simulink library "NeuroModelerLibrary"  (Simulink 10.2)
settings: Solver=ode45  StartTime=0.0  StopTime=10.0  RelTol=1e-3
libraries: $bdroot x672, simulink x5, neural x2
(part 4 of 5)

== system NeuroModelerLibrary/Sized Cells/CSNM4x3 ==
  Stimulate1 : Inport
  Stimulate2 : Inport  Port=2
  Stimulate3 : Inport  Port=3
  Stimulate4 : Inport  Port=4
  Arresting1 : Inport  Port=5
  Arresting2 : Inport  Port=6
  Arresting3 : Inport  Port=7
  Arresting4 : Inport  Port=8
  C1 : Constant
  C2 : Constant  Value=0.93
  C3 : Constant  Value=-1
  CSNM Compartment{,1..6} (7 alike) : $bdroot/Neuron Elements/CSNM Compartment  ACm=1e-9  ARm=1e7  ECm=1e-9  ERm=1e7  ARFm=1e7  ERFm=1e7  U0=-0.070  sign=-1
  CSNM LTZone : $bdroot/Neuron Elements/CSNM LTZone  NM=1  FB=2  T=-0.055  switchOff=-0.1
  CSNM Synapse{,1..7} (8 alike) : $bdroot/Neuron Elements/CSNM Synapse  SecretionTC=0.001  DecompositionTC=0.005  UseKsi=off  Rs=2e7  ksi=1  U0=-0.070  Weight=1  sign=off
  Sum7 : Sum  Inputs=++++++++  InputSameDT=on  SaturateOnIntegerOverflow=on  OutDataTypeStr=Inherit: Same as first input
  Out : Outport  VectorParamsAs1DForOutWhenUnconnected=off
  Visual : Outport  Port=2  VectorParamsAs1DForOutWhenUnconnected=off
  Potential : Outport  Port=3  VectorParamsAs1DForOutWhenUnconnected=off
  wires:
  CSNM Synapse7/1 -> CSNM Compartment/5
  Arresting4/1 -> CSNM Synapse7/1
  CSNM Synapse6/1 -> CSNM Compartment4/5
  Arresting3/1 -> CSNM Synapse6/1
  CSNM Synapse5/1 -> CSNM Compartment5/5
  Arresting2/1 -> CSNM Synapse5/1
  Stimulate4/1 -> CSNM Synapse/1
  CSNM Synapse/1 -> CSNM Compartment/1
  Stimulate3/1 -> CSNM Synapse1/1
  CSNM Synapse1/1 -> CSNM Compartment4/1
  Stimulate2/1 -> CSNM Synapse2/1
  CSNM Synapse2/1 -> CSNM Compartment5/1
  CSNM Synapse3/1 -> CSNM Compartment6/1
  CSNM Synapse4/1 -> CSNM Compartment6/5
  CSNM Compartment6/2 -> CSNM Compartment5/4
  CSNM Compartment6/1 -> CSNM Compartment5/2
  CSNM Compartment5/2 -> CSNM Compartment4/4
  CSNM Compartment5/1 -> CSNM Compartment4/2
  CSNM LTZone/4 -> Visual/1
  CSNM LTZone/1 -> Out/1
  C1/1 -> CSNM LTZone/2
  Stimulate1/1 -> CSNM Synapse3/1
  Arresting1/1 -> CSNM Synapse4/1
  C2/1 -> CSNM Compartment1/2, CSNM Compartment3/2, CSNM Compartment2/2, CSNM Compartment6/2
  C3/1 -> CSNM Compartment6/4, CSNM Compartment1/4, CSNM Compartment3/4, CSNM Compartment2/4
  Sum7/1 -> CSNM LTZone/1
  CSNM LTZone/3 -> CSNM Compartment/3, CSNM Compartment1/3, CSNM Compartment3/3, CSNM Compartment2/3
  CSNM Compartment/1 -> Sum7/1
  CSNM Compartment/2 -> Sum7/2
  CSNM LTZone/2 -> Potential/1
  CSNM Compartment1/1 -> Sum7/3
  CSNM Compartment1/2 -> Sum7/4
  CSNM Compartment2/1 -> Sum7/5
  CSNM Compartment2/2 -> Sum7/6
  CSNM Compartment3/1 -> Sum7/7
  CSNM Compartment3/2 -> Sum7/8
  CSNM Compartment4/2 -> CSNM Compartment/4
  CSNM Compartment4/1 -> CSNM Compartment/2

== system NeuroModelerLibrary/Sized Cells/Cell IaF 1x4 ==
  Stimulate1 : Inport
  Stimulate2 : Inport  Port=2
  Stimulate3 : Inport  Port=3
  Stimulate4 : Inport  Port=4
  CSNM Synapse{40..43} (4 alike) : $bdroot/Neuron Elements/CSNM Synapse  SecretionTC=0.001  DecompositionTC=0.005  UseKsi=off  Rs=2e7  ksi=1  U0=-0.070  Weight=1  sign=off
  Constant6 : Constant  Value=-0.070
  IaF LTZone6 : Subsystem  mask{tau_m=0.01, Cm=250e-12, I_const=0, E_L=-0.070, V_reset=-0.10, V_th=-0.055}
      mask prompts: tau_m "Membrane time constatnt"; Cm "Membrane capacity"; I_const "Constant input current"; E_L "Resting membrane potential"; V_reset "Reset membrane potential"; V_th "Threshold potential"
  IaF Membrane Segment18 : Subsystem  mask{tau_m=0.01, Cm=250e-12, I_const=0, E_L=-0.070, V_reset=-0.10, V_th=-0.055}
      mask prompts: tau_m "Membrane time constatnt"; Cm "Membrane capacity"; I_const "Constant input current"; E_L "Resting membrane potential"; V_reset "Reset membrane potential"; V_th "Threshold potential"
  IaF Membrane Segment19 : Subsystem  mask{tau_m=0.01, Cm=250e-12, I_const=0, E_L=-0.070, V_reset=-0.10, V_th=-0.055}
      mask prompts: tau_m "Membrane time constatnt"; Cm "Membrane capacity"; I_const "Constant input current"; E_L "Resting membrane potential"; V_reset "Reset membrane potential"; V_th "Threshold potential"
  IaF Membrane Segment20 : Subsystem  mask{tau_m=0.01, Cm=250e-12, I_const=0, E_L=-0.070, V_reset=-0.10, V_th=-0.055}
      mask prompts: tau_m "Membrane time constatnt"; Cm "Membrane capacity"; I_const "Constant input current"; E_L "Resting membrane potential"; V_reset "Reset membrane potential"; V_th "Threshold potential"
  IaF Membrane Segment21 : Subsystem  mask{tau_m=0.01, Cm=250e-12, I_const=0, E_L=-0.070, V_reset=-0.10, V_th=-0.055}
      mask prompts: tau_m "Membrane time constatnt"; Cm "Membrane capacity"; I_const "Constant input current"; E_L "Resting membrane potential"; V_reset "Reset membrane potential"; V_th "Threshold potential"
  Potential : Outport
  wires:
  IaF Membrane Segment21/1(Out1) -> IaF Membrane Segment20/2(Resting Potential)
  IaF Membrane Segment20/1(Out1) -> IaF Membrane Segment19/2(Resting Potential)
  IaF Membrane Segment19/1(Out1) -> IaF Membrane Segment18/2(Resting Potential)
  CSNM Synapse41/1 -> IaF Membrane Segment20/1(Synapses)
  IaF LTZone6/1(Out) -> IaF Membrane Segment18/3(Reset Signal)  "Out"
  IaF Membrane Segment18/1(Out1) -> IaF LTZone6/1(Potential)  "IaF синапс + IaF нейрон"
  Constant6/1 -> IaF Membrane Segment21/2(Resting Potential)
  CSNM Synapse40/1 -> IaF Membrane Segment21/1(Synapses)
  Stimulate4/1 -> CSNM Synapse40/1
  CSNM Synapse43/1 -> IaF Membrane Segment18/1(Synapses)
  CSNM Synapse42/1 -> IaF Membrane Segment19/1(Synapses)
  Stimulate3/1 -> CSNM Synapse41/1
  IaF LTZone6/2(Out Potential) -> Potential/1
  Stimulate1/1 -> CSNM Synapse43/1
  Stimulate2/1 -> CSNM Synapse42/1

== system NeuroModelerLibrary/Sized Cells/Cell IaF 1x4-Syn4 ==
  Stimulate1 : Inport
  Stimulate2 : Inport  Port=2
  Stimulate3 : Inport  Port=3
  Stimulate4 : Inport  Port=4
  CSNM Synapse{8..11} (4 alike) : $bdroot/Neuron Elements/CSNM Synapse  SecretionTC=0.001  DecompositionTC=0.005  UseKsi=off  Rs=2e7  ksi=1  U0=-0.070  Weight=1  sign=off
  Constant4 : Constant  Value=-0.070
  IaF LTZone1 : Subsystem  mask{tau_m=0.01, Cm=250e-12, I_const=0, E_L=-0.070, V_reset=-0.10, V_th=-0.055}
      mask prompts: tau_m "Membrane time constatnt"; Cm "Membrane capacity"; I_const "Constant input current"; E_L "Resting membrane potential"; V_reset "Reset membrane potential"; V_th "Threshold potential"
  IaF Membrane Segment1 : Subsystem  mask{tau_m=0.01, Cm=250e-12, I_const=0, E_L=-0.070, V_reset=-0.10, V_th=-0.055}
      mask prompts: tau_m "Membrane time constatnt"; Cm "Membrane capacity"; I_const "Constant input current"; E_L "Resting membrane potential"; V_reset "Reset membrane potential"; V_th "Threshold potential"
  IaF Membrane Segment2 : Subsystem  mask{tau_m=0.01, Cm=250e-12, I_const=0, E_L=-0.070, V_reset=-0.10, V_th=-0.055}
      mask prompts: tau_m "Membrane time constatnt"; Cm "Membrane capacity"; I_const "Constant input current"; E_L "Resting membrane potential"; V_reset "Reset membrane potential"; V_th "Threshold potential"
  IaF Membrane Segment3 : Subsystem  mask{tau_m=0.01, Cm=250e-12, I_const=0, E_L=-0.070, V_reset=-0.10, V_th=-0.055}
      mask prompts: tau_m "Membrane time constatnt"; Cm "Membrane capacity"; I_const "Constant input current"; E_L "Resting membrane potential"; V_reset "Reset membrane potential"; V_th "Threshold potential"
  IaF Membrane Segment4 : Subsystem  mask{tau_m=0.01, Cm=250e-12, I_const=0, E_L=-0.070, V_reset=-0.10, V_th=-0.055}
      mask prompts: tau_m "Membrane time constatnt"; Cm "Membrane capacity"; I_const "Constant input current"; E_L "Resting membrane potential"; V_reset "Reset membrane potential"; V_th "Threshold potential"
  Sum2 : Sum  Inputs=++++  InputSameDT=on  SaturateOnIntegerOverflow=on  OutDataTypeStr=Inherit: Same as first input
  Potential : Outport
  wires:
  Sum2/1 -> IaF Membrane Segment4/1(Synapses)
  CSNM Synapse8/1 -> Sum2/1
  CSNM Synapse9/1 -> Sum2/2
  IaF Membrane Segment4/1(Out1) -> IaF Membrane Segment3/2(Resting Potential)
  Stimulate1/1 -> CSNM Synapse8/1
  Constant4/1 -> IaF Membrane Segment4/2(Resting Potential)
  IaF Membrane Segment2/1(Out1) -> IaF Membrane Segment1/2(Resting Potential)
  CSNM Synapse10/1 -> Sum2/3
  IaF Membrane Segment1/1(Out1) -> IaF LTZone1/1(Potential)  "IaF синапс + IaF нейрон"
  CSNM Synapse11/1 -> Sum2/4
  IaF LTZone1/2(Out Potential) -> Potential/1  "1 syn"
  IaF Membrane Segment3/1(Out1) -> IaF Membrane Segment2/2(Resting Potential)
  IaF LTZone1/1(Out) -> IaF Membrane Segment1/3(Reset Signal)  "Out"
  Stimulate2/1 -> CSNM Synapse9/1
  Stimulate3/1 -> CSNM Synapse10/1
  Stimulate4/1 -> CSNM Synapse11/1

== system NeuroModelerLibrary/Sized Cells/Cell IaF 2x4 ==
  Stimulate1 : Inport
  Stimulate2 : Inport  Port=2
  Stimulate3 : Inport  Port=3
  Stimulate4 : Inport  Port=4
  CSNM Synapse{40..43} (4 alike) : $bdroot/Neuron Elements/CSNM Synapse  SecretionTC=0.001  DecompositionTC=0.005  UseKsi=off  Rs=2e7  ksi=1  U0=-0.070  Weight=1  sign=off
  Constant7 : Constant  Value=-0.070
  IaF LTZone7 : Subsystem  mask{tau_m=0.01, Cm=250e-12, I_const=0, E_L=-0.070, V_reset=-0.10, V_th=-0.055}
      mask prompts: tau_m "Membrane time constatnt"; Cm "Membrane capacity"; I_const "Constant input current"; E_L "Resting membrane potential"; V_reset "Reset membrane potential"; V_th "Threshold potential"
  IaF Membrane Segment22 : Subsystem  mask{tau_m=0.01, Cm=250e-12, I_const=0, E_L=-0.070, V_reset=-0.10, V_th=-0.055}
      mask prompts: tau_m "Membrane time constatnt"; Cm "Membrane capacity"; I_const "Constant input current"; E_L "Resting membrane potential"; V_reset "Reset membrane potential"; V_th "Threshold potential"
  IaF Membrane Segment23 : Subsystem  mask{tau_m=0.01, Cm=250e-12, I_const=0, E_L=-0.070, V_reset=-0.10, V_th=-0.055}
      mask prompts: tau_m "Membrane time constatnt"; Cm "Membrane capacity"; I_const "Constant input current"; E_L "Resting membrane potential"; V_reset "Reset membrane potential"; V_th "Threshold potential"
  IaF Membrane Segment24 : Subsystem  mask{tau_m=0.01, Cm=250e-12, I_const=0, E_L=-0.070, V_reset=-0.10, V_th=-0.055}
      mask prompts: tau_m "Membrane time constatnt"; Cm "Membrane capacity"; I_const "Constant input current"; E_L "Resting membrane potential"; V_reset "Reset membrane potential"; V_th "Threshold potential"
  IaF Membrane Segment25 : Subsystem  mask{tau_m=0.01, Cm=250e-12, I_const=0, E_L=-0.070, V_reset=-0.10, V_th=-0.055}
      mask prompts: tau_m "Membrane time constatnt"; Cm "Membrane capacity"; I_const "Constant input current"; E_L "Resting membrane potential"; V_reset "Reset membrane potential"; V_th "Threshold potential"
  IaF Membrane Segment26 : Subsystem  mask{tau_m=0.01, Cm=250e-12, I_const=0, E_L=-0.070, V_reset=-0.10, V_th=-0.055}
      mask prompts: tau_m "Membrane time constatnt"; Cm "Membrane capacity"; I_const "Constant input current"; E_L "Resting membrane potential"; V_reset "Reset membrane potential"; V_th "Threshold potential"
  Sum : Sum  Inputs=|++
  Potential : Outport
  wires:
  IaF LTZone7/1(Out) -> IaF Membrane Segment26/3(Reset Signal), IaF Membrane Segment22/3(Reset Signal)  "Out"
  Constant7/1 -> IaF Membrane Segment25/2(Resting Potential), IaF Membrane Segment26/2(Resting Potential)
  IaF Membrane Segment24/1(Out1) -> IaF Membrane Segment23/2(Resting Potential)
  IaF Membrane Segment22/1(Out1) -> Sum/1
  IaF Membrane Segment25/1(Out1) -> IaF Membrane Segment24/2(Resting Potential)
  Sum/1 -> IaF LTZone7/1(Potential)
  IaF Membrane Segment26/1(Out1) -> Sum/2
  IaF Membrane Segment23/1(Out1) -> IaF Membrane Segment22/2(Resting Potential)
  IaF LTZone7/2(Out Potential) -> Potential/1
  Stimulate3/1 -> CSNM Synapse41/1
  Stimulate4/1 -> CSNM Synapse40/1
  CSNM Synapse43/1 -> IaF Membrane Segment22/1(Synapses)
  CSNM Synapse42/1 -> IaF Membrane Segment23/1(Synapses)
  CSNM Synapse40/1 -> IaF Membrane Segment25/1(Synapses)
  Stimulate1/1 -> CSNM Synapse43/1
  CSNM Synapse41/1 -> IaF Membrane Segment24/1(Synapses)
  Stimulate2/1 -> CSNM Synapse42/1

== system NeuroModelerLibrary/Sized Cells/Cell IaF 3x4 ==
  Stimulate1 : Inport
  Stimulate2 : Inport  Port=2
  Stimulate3 : Inport  Port=3
  Stimulate4 : Inport  Port=4
  CSNM Synapse{40..43} (4 alike) : $bdroot/Neuron Elements/CSNM Synapse  SecretionTC=0.001  DecompositionTC=0.005  UseKsi=off  Rs=2e7  ksi=1  U0=-0.070  Weight=1  sign=off
  Constant8 : Constant  Value=-0.070
  IaF LTZone8 : Subsystem  mask{tau_m=0.01, Cm=250e-12, I_const=0, E_L=-0.070, V_reset=-0.10, V_th=-0.055}
      mask prompts: tau_m "Membrane time constatnt"; Cm "Membrane capacity"; I_const "Constant input current"; E_L "Resting membrane potential"; V_reset "Reset membrane potential"; V_th "Threshold potential"
  IaF Membrane Segment27 : Subsystem  mask{tau_m=0.01, Cm=250e-12, I_const=0, E_L=-0.070, V_reset=-0.10, V_th=-0.055}
      mask prompts: tau_m "Membrane time constatnt"; Cm "Membrane capacity"; I_const "Constant input current"; E_L "Resting membrane potential"; V_reset "Reset membrane potential"; V_th "Threshold potential"
  IaF Membrane Segment28 : Subsystem  mask{tau_m=0.01, Cm=250e-12, I_const=0, E_L=-0.070, V_reset=-0.10, V_th=-0.055}
      mask prompts: tau_m "Membrane time constatnt"; Cm "Membrane capacity"; I_const "Constant input current"; E_L "Resting membrane potential"; V_reset "Reset membrane potential"; V_th "Threshold potential"
  IaF Membrane Segment29 : Subsystem  mask{tau_m=0.01, Cm=250e-12, I_const=0, E_L=-0.070, V_reset=-0.10, V_th=-0.055}
      mask prompts: tau_m "Membrane time constatnt"; Cm "Membrane capacity"; I_const "Constant input current"; E_L "Resting membrane potential"; V_reset "Reset membrane potential"; V_th "Threshold potential"
  IaF Membrane Segment30 : Subsystem  mask{tau_m=0.01, Cm=250e-12, I_const=0, E_L=-0.070, V_reset=-0.10, V_th=-0.055}
      mask prompts: tau_m "Membrane time constatnt"; Cm "Membrane capacity"; I_const "Constant input current"; E_L "Resting membrane potential"; V_reset "Reset membrane potential"; V_th "Threshold potential"
  IaF Membrane Segment31 : Subsystem  mask{tau_m=0.01, Cm=250e-12, I_const=0, E_L=-0.070, V_reset=-0.10, V_th=-0.055}
      mask prompts: tau_m "Membrane time constatnt"; Cm "Membrane capacity"; I_const "Constant input current"; E_L "Resting membrane potential"; V_reset "Reset membrane potential"; V_th "Threshold potential"
  IaF Membrane Segment32 : Subsystem  mask{tau_m=0.01, Cm=250e-12, I_const=0, E_L=-0.070, V_reset=-0.10, V_th=-0.055}
      mask prompts: tau_m "Membrane time constatnt"; Cm "Membrane capacity"; I_const "Constant input current"; E_L "Resting membrane potential"; V_reset "Reset membrane potential"; V_th "Threshold potential"
  Sum10 : Sum  Inputs=|+++
  Potential : Outport
  wires:
  IaF Membrane Segment31/1(Out1) -> Sum10/2
  IaF LTZone8/1(Out) -> IaF Membrane Segment32/3(Reset Signal), IaF Membrane Segment31/3(Reset Signal), IaF Membrane Segment27/3(Reset Signal)  "Out"
  IaF Membrane Segment30/1(Out1) -> IaF Membrane Segment29/2(Resting Potential)
  IaF Membrane Segment27/1(Out1) -> Sum10/1
  IaF Membrane Segment29/1(Out1) -> IaF Membrane Segment28/2(Resting Potential)
  Sum10/1 -> IaF LTZone8/1(Potential)
  IaF Membrane Segment32/1(Out1) -> Sum10/3
  IaF Membrane Segment28/1(Out1) -> IaF Membrane Segment27/2(Resting Potential)
  Constant8/1 -> IaF Membrane Segment30/2(Resting Potential), IaF Membrane Segment32/2(Resting Potential), IaF Membrane Segment31/2(Resting Potential)
  IaF LTZone8/2(Out Potential) -> Potential/1
  Stimulate3/1 -> CSNM Synapse41/1
  Stimulate4/1 -> CSNM Synapse40/1
  CSNM Synapse43/1 -> IaF Membrane Segment27/1(Synapses)
  CSNM Synapse42/1 -> IaF Membrane Segment28/1(Synapses)
  CSNM Synapse40/1 -> IaF Membrane Segment30/1(Synapses)
  Stimulate1/1 -> CSNM Synapse43/1
  CSNM Synapse41/1 -> IaF Membrane Segment29/1(Synapses)
  Stimulate2/1 -> CSNM Synapse42/1

== system NeuroModelerLibrary/Sized Cells/Cell IaF 4x4 ==
  Stimulate1 : Inport
  Stimulate2 : Inport  Port=2
  Stimulate3 : Inport  Port=3
  Stimulate4 : Inport  Port=4
  CSNM Synapse{40..43} (4 alike) : $bdroot/Neuron Elements/CSNM Synapse  SecretionTC=0.001  DecompositionTC=0.005  UseKsi=off  Rs=2e7  ksi=1  U0=-0.070  Weight=1  sign=off
  Constant9 : Constant  Value=-0.070
  IaF LTZone9 : Subsystem  mask{tau_m=0.01, Cm=250e-12, I_const=0, E_L=-0.070, V_reset=-0.10, V_th=-0.055}
      mask prompts: tau_m "Membrane time constatnt"; Cm "Membrane capacity"; I_const "Constant input current"; E_L "Resting membrane potential"; V_reset "Reset membrane potential"; V_th "Threshold potential"
  IaF Membrane Segment33 : Subsystem  mask{tau_m=0.01, Cm=250e-12, I_const=0, E_L=-0.070, V_reset=-0.10, V_th=-0.055}
      mask prompts: tau_m "Membrane time constatnt"; Cm "Membrane capacity"; I_const "Constant input current"; E_L "Resting membrane potential"; V_reset "Reset membrane potential"; V_th "Threshold potential"
  IaF Membrane Segment34 : Subsystem  mask{tau_m=0.01, Cm=250e-12, I_const=0, E_L=-0.070, V_reset=-0.10, V_th=-0.055}
      mask prompts: tau_m "Membrane time constatnt"; Cm "Membrane capacity"; I_const "Constant input current"; E_L "Resting membrane potential"; V_reset "Reset membrane potential"; V_th "Threshold potential"
  IaF Membrane Segment35 : Subsystem  mask{tau_m=0.01, Cm=250e-12, I_const=0, E_L=-0.070, V_reset=-0.10, V_th=-0.055}
      mask prompts: tau_m "Membrane time constatnt"; Cm "Membrane capacity"; I_const "Constant input current"; E_L "Resting membrane potential"; V_reset "Reset membrane potential"; V_th "Threshold potential"
  IaF Membrane Segment36 : Subsystem  mask{tau_m=0.01, Cm=250e-12, I_const=0, E_L=-0.070, V_reset=-0.10, V_th=-0.055}
      mask prompts: tau_m "Membrane time constatnt"; Cm "Membrane capacity"; I_const "Constant input current"; E_L "Resting membrane potential"; V_reset "Reset membrane potential"; V_th "Threshold potential"
  IaF Membrane Segment37 : Subsystem  mask{tau_m=0.01, Cm=250e-12, I_const=0, E_L=-0.070, V_reset=-0.10, V_th=-0.055}
      mask prompts: tau_m "Membrane time constatnt"; Cm "Membrane capacity"; I_const "Constant input current"; E_L "Resting membrane potential"; V_reset "Reset membrane potential"; V_th "Threshold potential"
  IaF Membrane Segment38 : Subsystem  mask{tau_m=0.01, Cm=250e-12, I_const=0, E_L=-0.070, V_reset=-0.10, V_th=-0.055}
      mask prompts: tau_m "Membrane time constatnt"; Cm "Membrane capacity"; I_const "Constant input current"; E_L "Resting membrane potential"; V_reset "Reset membrane potential"; V_th "Threshold potential"
  IaF Membrane Segment39 : Subsystem  mask{tau_m=0.01, Cm=250e-12, I_const=0, E_L=-0.070, V_reset=-0.10, V_th=-0.055}
      mask prompts: tau_m "Membrane time constatnt"; Cm "Membrane capacity"; I_const "Constant input current"; E_L "Resting membrane potential"; V_reset "Reset membrane potential"; V_th "Threshold potential"
  Sum11 : Sum  Inputs=|++++
  Potential : Outport
  wires:
  Constant9/1 -> IaF Membrane Segment36/2(Resting Potential), IaF Membrane Segment39/2(Resting Potential), IaF Membrane Segment38/2(Resting Potential), IaF Membrane Segment37/2(Resting Potential)
  IaF LTZone9/1(Out) -> IaF Membrane Segment39/3(Reset Signal), IaF Membrane Segment38/3(Reset Signal), IaF Membrane Segment37/3(Reset Signal), IaF Membrane Segment33/3(Reset Signal)  "Out"
  IaF Membrane Segment36/1(Out1) -> IaF Membrane Segment35/2(Resting Potential)
  IaF Membrane Segment33/1(Out1) -> Sum11/1
  IaF Membrane Segment39/1(Out1) -> Sum11/4
  IaF LTZone9/2(Out Potential) -> Potential/1
  IaF Membrane Segment38/1(Out1) -> Sum11/3
  Sum11/1 -> IaF LTZone9/1(Potential)
  IaF Membrane Segment37/1(Out1) -> Sum11/2
  IaF Membrane Segment35/1(Out1) -> IaF Membrane Segment34/2(Resting Potential)
  IaF Membrane Segment34/1(Out1) -> IaF Membrane Segment33/2(Resting Potential)
  Stimulate3/1 -> CSNM Synapse41/1
  Stimulate4/1 -> CSNM Synapse40/1
  CSNM Synapse43/1 -> IaF Membrane Segment33/1(Synapses)
  CSNM Synapse42/1 -> IaF Membrane Segment34/1(Synapses)
  CSNM Synapse40/1 -> IaF Membrane Segment36/1(Synapses)
  Stimulate1/1 -> CSNM Synapse43/1
  CSNM Synapse41/1 -> IaF Membrane Segment35/1(Synapses)
  Stimulate2/1 -> CSNM Synapse42/1

== system NeuroModelerLibrary/Sized Cells/Size Cell ==
  Stimulate1 : Inport
  Stimulate2 : Inport  Port=2
  Stimulate3 : Inport  Port=3
  Stimulate4 : Inport  Port=4
  Arresting1 : Inport  Port=5
  Arresting2 : Inport  Port=6
  Arresting3 : Inport  Port=7
  Arresting4 : Inport  Port=8
  C1 : Constant
  C2 : Constant
  C3 : Constant  Value=-1
  LTZone : $bdroot/Neuron Elements/LTZone  NM=1  FB=1.7  IT=0.005  T=0.001
  Simple Membrane{,1..3} (4 alike) : $bdroot/Neuron Elements/Simple Membrane  ACm=1e-9  ARm=1e7  ECm=1e-9  ERm=1e7  ARFm=1e8  ERFm=1e8
  Sum12 : Sum  InputSameDT=on  SaturateOnIntegerOverflow=on  OutDataTypeStr=Inherit: Same as first input
  Sum7 : Sum  InputSameDT=on  SaturateOnIntegerOverflow=on  OutDataTypeStr=Inherit: Same as first input
  Synapse{,1..7} (8 alike) : $bdroot/Neuron Elements/Synapse  SecretionTC=0.001  DecompositionTC=0.01  UseKsi=on  ksi=2  gamma=1e8
  Out : Outport  VectorParamsAs1DForOutWhenUnconnected=off
  Visual : Outport  Port=2  VectorParamsAs1DForOutWhenUnconnected=off
  Potential : Outport  Port=3  VectorParamsAs1DForOutWhenUnconnected=off
  wires:
  Synapse7/1 -> Simple Membrane/5
  Arresting4/1 -> Synapse7/1
  Synapse6/1 -> Simple Membrane1/5
  Arresting3/1 -> Synapse6/1
  Synapse5/1 -> Simple Membrane2/5
  Arresting2/1 -> Synapse5/1
  Stimulate4/1 -> Synapse/1
  Synapse/1 -> Simple Membrane/1
  Stimulate3/1 -> Synapse2/1
  Synapse2/1 -> Simple Membrane1/1
  Stimulate2/1 -> Synapse3/1
  Synapse3/1 -> Simple Membrane2/1
  Synapse4/1 -> Simple Membrane3/1
  C2/1 -> Simple Membrane3/2
  C3/1 -> Simple Membrane3/4
  Synapse1/1 -> Simple Membrane3/5
  Simple Membrane3/2 -> Simple Membrane2/4
  Simple Membrane3/1 -> Simple Membrane2/2
  Simple Membrane2/2 -> Simple Membrane1/4
  Simple Membrane2/1 -> Simple Membrane1/2
  LTZone/2 -> Visual/1
  LTZone/3 -> Out/1
  C1/1 -> LTZone/2
  Stimulate1/1 -> Synapse4/1
  Arresting1/1 -> Synapse1/1
  Simple Membrane1/1 -> Sum12/1, Simple Membrane/2
  Simple Membrane1/2 -> Sum12/2, Simple Membrane/4
  Sum7/1 -> Potential/1, LTZone/1
  LTZone/1 -> Simple Membrane/3
  Simple Membrane/1 -> Sum7/1
  Simple Membrane/2 -> Sum7/2

== system NeuroModelerLibrary/Sized Cells/Size2 Cell ==
  Stimulate1 : Inport
  Stimulate2 : Inport  Port=2
  Stimulate3 : Inport  Port=3
  Stimulate4 : Inport  Port=4
  Arresting1 : Inport  Port=5
  Arresting2 : Inport  Port=6
  Arresting3 : Inport  Port=7
  Arresting4 : Inport  Port=8
  C1 : Constant
  C2 : Constant
  C3 : Constant  Value=-1
  C4 : Constant
  C5 : Constant  Value=-1
  LTZone : $bdroot/Neuron Elements/LTZone  NM=2  FB=1.2  IT=0.005  T=0.001
  Simple Membrane{,1..4} (5 alike) : $bdroot/Neuron Elements/Simple Membrane  ACm=1e-9  ARm=1e7  ECm=1e-9  ERm=1e7  ARFm=1e8  ERFm=1e8
  Sum1 : Sum  InputSameDT=on  SaturateOnIntegerOverflow=on  OutDataTypeStr=Inherit: Same as first input
  Sum12 : Sum  InputSameDT=on  SaturateOnIntegerOverflow=on  OutDataTypeStr=Inherit: Same as first input
  Sum7 : Sum  Inputs=++++  InputSameDT=on  SaturateOnIntegerOverflow=on  OutDataTypeStr=Inherit: Same as first input
  Synapse{,1..7} (8 alike) : $bdroot/Neuron Elements/Synapse  SecretionTC=0.001  DecompositionTC=0.01  UseKsi=on  ksi=2  gamma=1e8
  Out : Outport  VectorParamsAs1DForOutWhenUnconnected=off
  Visual : Outport  Port=2  VectorParamsAs1DForOutWhenUnconnected=off
  Potential : Outport  Port=3  VectorParamsAs1DForOutWhenUnconnected=off
  wires:
  Synapse7/1 -> Simple Membrane/5
  Arresting4/1 -> Synapse7/1
  Synapse6/1 -> Simple Membrane1/5
  Arresting3/1 -> Synapse6/1
  Synapse5/1 -> Simple Membrane2/5
  Arresting2/1 -> Synapse5/1
  Stimulate4/1 -> Synapse4/1
  Synapse4/1 -> Simple Membrane/1
  Stimulate3/1 -> Synapse3/1
  Synapse3/1 -> Simple Membrane1/1
  Stimulate2/1 -> Synapse2/1
  Synapse2/1 -> Simple Membrane2/1
  Synapse/1 -> Simple Membrane3/1
  C2/1 -> Simple Membrane3/2
  C3/1 -> Simple Membrane3/4
  Synapse1/1 -> Simple Membrane3/5
  Simple Membrane3/2 -> Simple Membrane2/4
  Simple Membrane3/1 -> Simple Membrane2/2
  Simple Membrane2/2 -> Simple Membrane1/4
  Simple Membrane2/1 -> Simple Membrane1/2
  LTZone/2 -> Visual/1
  LTZone/3 -> Out/1
  C1/1 -> LTZone/2
  Stimulate1/1 -> Synapse/1
  Arresting1/1 -> Synapse1/1
  Simple Membrane1/1 -> Sum12/1, Simple Membrane/2
  Simple Membrane1/2 -> Sum12/2, Simple Membrane/4
  Sum7/1 -> LTZone/1, Potential/1
  LTZone/1 -> Simple Membrane/3, Simple Membrane4/3
  Simple Membrane4/1 -> Sum1/1
  Simple Membrane4/2 -> Sum1/2
  Sum1/1 -> Sum7/1
  Simple Membrane/2 -> Sum7/3
  Simple Membrane/1 -> Sum7/2
  C4/1 -> Simple Membrane4/2
  C5/1 -> Simple Membrane4/4

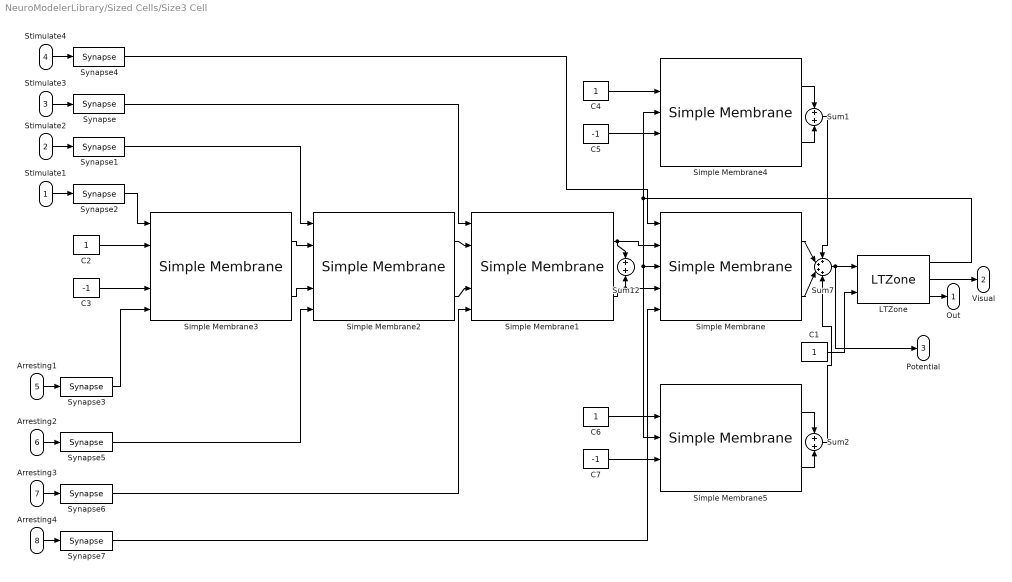
== system NeuroModelerLibrary/Sized Cells/Size3 Cell ==
  Stimulate1 : Inport
  Stimulate2 : Inport  Port=2
  Stimulate3 : Inport  Port=3
  Stimulate4 : Inport  Port=4
  Arresting1 : Inport  Port=5
  Arresting2 : Inport  Port=6
  Arresting3 : Inport  Port=7
  Arresting4 : Inport  Port=8
  C{1..2,4,6} (4 alike) : Constant
  C3 : Constant  Value=-1
  C5 : Constant  Value=-1
  C7 : Constant  Value=-1
  LTZone : $bdroot/Neuron Elements/LTZone  NM=3  FB=1  IT=0.005  T=0.001
  Simple Membrane{,1..5} (6 alike) : $bdroot/Neuron Elements/Simple Membrane  ACm=1e-9  ARm=1e7  ECm=1e-9  ERm=1e7  ARFm=1e8  ERFm=1e8
  Sum1 : Sum  InputSameDT=on  SaturateOnIntegerOverflow=on  OutDataTypeStr=Inherit: Same as first input
  Sum12 : Sum  InputSameDT=on  SaturateOnIntegerOverflow=on  OutDataTypeStr=Inherit: Same as first input
  Sum2 : Sum  InputSameDT=on  SaturateOnIntegerOverflow=on  OutDataTypeStr=Inherit: Same as first input
  Sum7 : Sum  Inputs=++++  InputSameDT=on  SaturateOnIntegerOverflow=on  OutDataTypeStr=Inherit: Same as first input
  Synapse{,1..7} (8 alike) : $bdroot/Neuron Elements/Synapse  SecretionTC=0.001  DecompositionTC=0.01  UseKsi=on  ksi=2  gamma=1e8
  Out : Outport  VectorParamsAs1DForOutWhenUnconnected=off
  Visual : Outport  Port=2  VectorParamsAs1DForOutWhenUnconnected=off
  Potential : Outport  Port=3  VectorParamsAs1DForOutWhenUnconnected=off
  wires:
  C5/1 -> Simple Membrane4/4
  C4/1 -> Simple Membrane4/2
  Simple Membrane/1 -> Sum7/2
  Simple Membrane/2 -> Sum7/3
  Sum1/1 -> Sum7/1
  Simple Membrane4/2 -> Sum1/2
  Simple Membrane4/1 -> Sum1/1
  LTZone/1 -> Simple Membrane/3, Simple Membrane5/3, Simple Membrane4/3
  Sum7/1 -> LTZone/1, Potential/1
  Simple Membrane1/2 -> Sum12/2, Simple Membrane/4
  Simple Membrane1/1 -> Sum12/1, Simple Membrane/2
  Arresting1/1 -> Synapse3/1
  Stimulate1/1 -> Synapse2/1
  C1/1 -> LTZone/2
  LTZone/3 -> Out/1
  LTZone/2 -> Visual/1
  Simple Membrane2/1 -> Simple Membrane1/2
  Simple Membrane2/2 -> Simple Membrane1/4
  Simple Membrane3/1 -> Simple Membrane2/2
  Simple Membrane3/2 -> Simple Membrane2/4
  Synapse3/1 -> Simple Membrane3/5
  C3/1 -> Simple Membrane3/4
  C2/1 -> Simple Membrane3/2
  Synapse2/1 -> Simple Membrane3/1
  Synapse1/1 -> Simple Membrane2/1
  Stimulate2/1 -> Synapse1/1
  Synapse/1 -> Simple Membrane1/1
  Stimulate3/1 -> Synapse/1
  Synapse4/1 -> Simple Membrane/1
  Stimulate4/1 -> Synapse4/1
  Arresting2/1 -> Synapse5/1
  Synapse5/1 -> Simple Membrane2/5
  Arresting3/1 -> Synapse6/1
  Synapse6/1 -> Simple Membrane1/5
  Arresting4/1 -> Synapse7/1
  Synapse7/1 -> Simple Membrane/5
  C7/1 -> Simple Membrane5/4
  C6/1 -> Simple Membrane5/2
  Simple Membrane5/2 -> Sum2/2
  Simple Membrane5/1 -> Sum2/1
  Sum2/1 -> Sum7/4

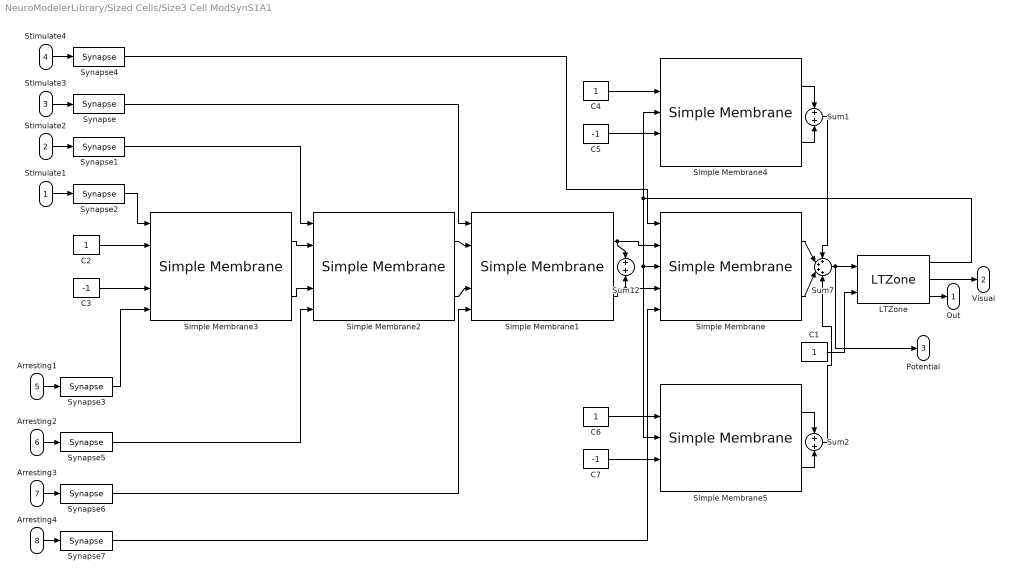
== system NeuroModelerLibrary/Sized Cells/Size3 Cell ModSynS1A1 ==
  Stimulate1 : Inport
  Stimulate2 : Inport  Port=2
  Stimulate3 : Inport  Port=3
  Stimulate4 : Inport  Port=4
  Arresting1 : Inport  Port=5
  Arresting2 : Inport  Port=6
  Arresting3 : Inport  Port=7
  Arresting4 : Inport  Port=8
  C{1..2,4,6} (4 alike) : Constant
  C3 : Constant  Value=-1
  C5 : Constant  Value=-1
  C7 : Constant  Value=-1
  LTZone : $bdroot/Neuron Elements/LTZone  NM=3  FB=1  IT=0.005  T=0.001
  Simple Membrane{,1..5} (6 alike) : $bdroot/Neuron Elements/Simple Membrane  ACm=1e-9  ARm=1e7  ECm=1e-9  ERm=1e7  ARFm=1e8  ERFm=1e8
  Sum1 : Sum  InputSameDT=on  SaturateOnIntegerOverflow=on  OutDataTypeStr=Inherit: Same as first input
  Sum12 : Sum  InputSameDT=on  SaturateOnIntegerOverflow=on  OutDataTypeStr=Inherit: Same as first input
  Sum2 : Sum  InputSameDT=on  SaturateOnIntegerOverflow=on  OutDataTypeStr=Inherit: Same as first input
  Sum7 : Sum  Inputs=++++  InputSameDT=on  SaturateOnIntegerOverflow=on  OutDataTypeStr=Inherit: Same as first input
  Synapse{,1,4..7} (6 alike) : $bdroot/Neuron Elements/Synapse  SecretionTC=0.001  DecompositionTC=0.01  UseKsi=on  ksi=2  gamma=1e8
  Synapse2 : $bdroot/Neuron Elements/Synapse  SecretionTC=0.001  DecompositionTC=0.01  UseKsi=on  ksi=1  gamma=1e8
  Synapse3 : $bdroot/Neuron Elements/Synapse  SecretionTC=0.001  DecompositionTC=0.01  UseKsi=on  ksi=1  gamma=1e8
  Out : Outport  VectorParamsAs1DForOutWhenUnconnected=off
  Visual : Outport  Port=2  VectorParamsAs1DForOutWhenUnconnected=off
  Potential : Outport  Port=3  VectorParamsAs1DForOutWhenUnconnected=off
  wires:
  C5/1 -> Simple Membrane4/4
  C4/1 -> Simple Membrane4/2
  Simple Membrane/1 -> Sum7/2
  Simple Membrane/2 -> Sum7/3
  Sum1/1 -> Sum7/1
  Simple Membrane4/2 -> Sum1/2
  Simple Membrane4/1 -> Sum1/1
  LTZone/1 -> Simple Membrane/3, Simple Membrane5/3, Simple Membrane4/3
  Sum7/1 -> LTZone/1, Potential/1
  Simple Membrane1/2 -> Sum12/2, Simple Membrane/4
  Simple Membrane1/1 -> Sum12/1, Simple Membrane/2
  Arresting1/1 -> Synapse3/1
  Stimulate1/1 -> Synapse2/1
  C1/1 -> LTZone/2
  LTZone/3 -> Out/1
  LTZone/2 -> Visual/1
  Simple Membrane2/1 -> Simple Membrane1/2
  Simple Membrane2/2 -> Simple Membrane1/4
  Simple Membrane3/1 -> Simple Membrane2/2
  Simple Membrane3/2 -> Simple Membrane2/4
  Synapse3/1 -> Simple Membrane3/5
  C3/1 -> Simple Membrane3/4
  C2/1 -> Simple Membrane3/2
  Synapse2/1 -> Simple Membrane3/1
  Synapse1/1 -> Simple Membrane2/1
  Stimulate2/1 -> Synapse1/1
  Synapse/1 -> Simple Membrane1/1
  Stimulate3/1 -> Synapse/1
  Synapse4/1 -> Simple Membrane/1
  Stimulate4/1 -> Synapse4/1
  Arresting2/1 -> Synapse5/1
  Synapse5/1 -> Simple Membrane2/5
  Arresting3/1 -> Synapse6/1
  Synapse6/1 -> Simple Membrane1/5
  Arresting4/1 -> Synapse7/1
  Synapse7/1 -> Simple Membrane/5
  C7/1 -> Simple Membrane5/4
  C6/1 -> Simple Membrane5/2
  Simple Membrane5/2 -> Sum2/2
  Simple Membrane5/1 -> Sum2/1
  Sum2/1 -> Sum7/4

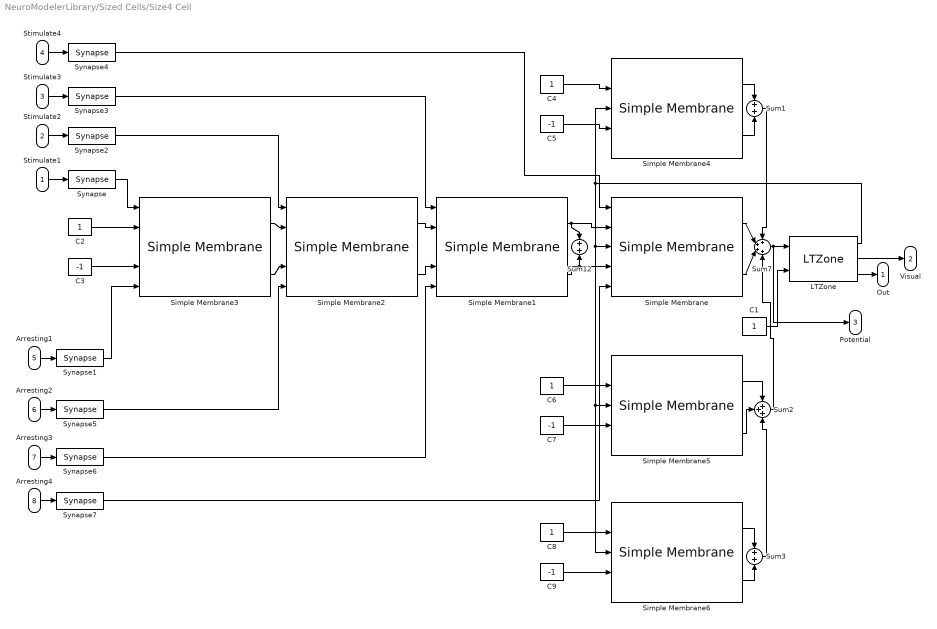
== system NeuroModelerLibrary/Sized Cells/Size4 Cell ==
  Stimulate1 : Inport
  Stimulate2 : Inport  Port=2
  Stimulate3 : Inport  Port=3
  Stimulate4 : Inport  Port=4
  Arresting1 : Inport  Port=5
  Arresting2 : Inport  Port=6
  Arresting3 : Inport  Port=7
  Arresting4 : Inport  Port=8
  C{1..2,4,6,8} (5 alike) : Constant
  C{3,5,7,9} (4 alike) : Constant  Value=-1
  LTZone : $bdroot/Neuron Elements/LTZone  NM=4  FB=0.9  IT=0.005  T=0.001
  Simple Membrane{,1..6} (7 alike) : $bdroot/Neuron Elements/Simple Membrane  ACm=1e-9  ARm=1e7  ECm=1e-9  ERm=1e7  ARFm=1e8  ERFm=1e8
  Sum1 : Sum  InputSameDT=on  SaturateOnIntegerOverflow=on  OutDataTypeStr=Inherit: Same as first input
  Sum12 : Sum  InputSameDT=on  SaturateOnIntegerOverflow=on  OutDataTypeStr=Inherit: Same as first input
  Sum2 : Sum  Inputs=+++  InputSameDT=on  SaturateOnIntegerOverflow=on  OutDataTypeStr=Inherit: Same as first input
  Sum3 : Sum  InputSameDT=on  SaturateOnIntegerOverflow=on  OutDataTypeStr=Inherit: Same as first input
  Sum7 : Sum  Inputs=++++  InputSameDT=on  SaturateOnIntegerOverflow=on  OutDataTypeStr=Inherit: Same as first input
  Synapse{,1..7} (8 alike) : $bdroot/Neuron Elements/Synapse  SecretionTC=0.001  DecompositionTC=0.01  UseKsi=on  ksi=2  gamma=1e8
  Out : Outport  VectorParamsAs1DForOutWhenUnconnected=off
  Visual : Outport  Port=2  VectorParamsAs1DForOutWhenUnconnected=off
  Potential : Outport  Port=3  VectorParamsAs1DForOutWhenUnconnected=off
  wires:
  Sum2/1 -> Sum7/4
  Simple Membrane5/1 -> Sum2/1
  C6/1 -> Simple Membrane5/2
  C7/1 -> Simple Membrane5/4
  Synapse7/1 -> Simple Membrane/5
  Arresting4/1 -> Synapse7/1
  Synapse6/1 -> Simple Membrane1/5
  Arresting3/1 -> Synapse6/1
  Synapse5/1 -> Simple Membrane2/5
  Arresting2/1 -> Synapse5/1
  Stimulate4/1 -> Synapse4/1
  Synapse4/1 -> Simple Membrane/1
  Stimulate3/1 -> Synapse3/1
  Synapse3/1 -> Simple Membrane1/1
  Stimulate2/1 -> Synapse2/1
  Synapse2/1 -> Simple Membrane2/1
  Synapse/1 -> Simple Membrane3/1
  C2/1 -> Simple Membrane3/2
  C3/1 -> Simple Membrane3/4
  Synapse1/1 -> Simple Membrane3/5
  Simple Membrane3/2 -> Simple Membrane2/4
  Simple Membrane3/1 -> Simple Membrane2/2
  Simple Membrane2/2 -> Simple Membrane1/4
  Simple Membrane2/1 -> Simple Membrane1/2
  LTZone/2 -> Visual/1
  LTZone/3 -> Out/1
  C1/1 -> LTZone/2
  Stimulate1/1 -> Synapse/1
  Arresting1/1 -> Synapse1/1
  Simple Membrane1/1 -> Sum12/1, Simple Membrane/2
  Simple Membrane1/2 -> Sum12/2, Simple Membrane/4
  Sum7/1 -> LTZone/1, Potential/1
  LTZone/1 -> Simple Membrane5/3, Simple Membrane6/3, Simple Membrane/3, Simple Membrane4/3
  Simple Membrane4/1 -> Sum1/1
  Simple Membrane4/2 -> Sum1/2
  Sum1/1 -> Sum7/1
  Simple Membrane/2 -> Sum7/3
  Simple Membrane/1 -> Sum7/2
  C4/1 -> Simple Membrane4/2
  C5/1 -> Simple Membrane4/4
  Simple Membrane6/1 -> Sum3/1
  Simple Membrane6/2 -> Sum3/2
  C8/1 -> Simple Membrane6/2
  C9/1 -> Simple Membrane6/4
  Sum3/1 -> Sum2/3
  Simple Membrane5/2 -> Sum2/2

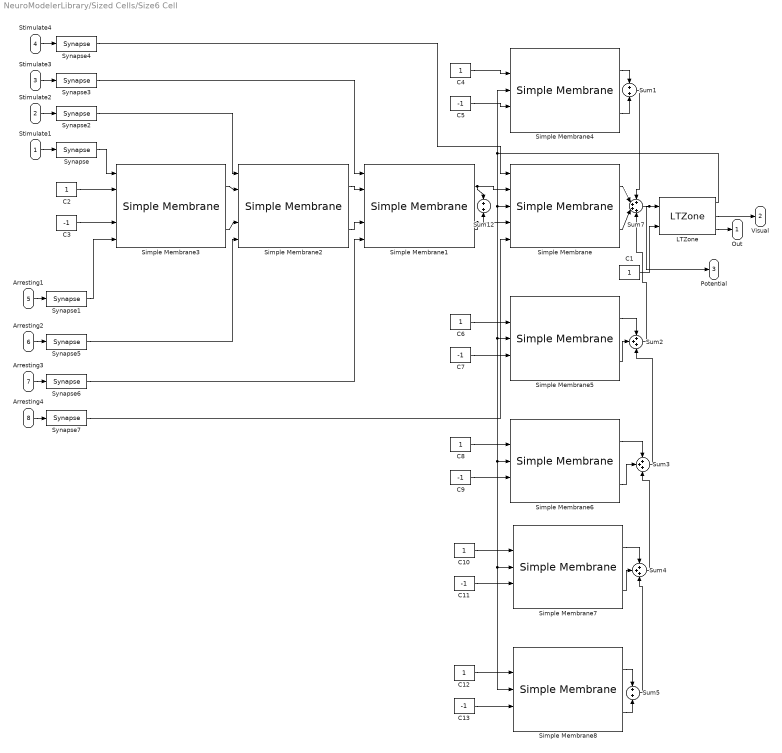
== system NeuroModelerLibrary/Sized Cells/Size6 Cell ==
  Stimulate1 : Inport
  Stimulate2 : Inport  Port=2
  Stimulate3 : Inport  Port=3
  Stimulate4 : Inport  Port=4
  Arresting1 : Inport  Port=5
  Arresting2 : Inport  Port=6
  Arresting3 : Inport  Port=7
  Arresting4 : Inport  Port=8
  C{1..2,4,6,8,10,12} (7 alike) : Constant
  C{3,5,7,9,11,13} (6 alike) : Constant  Value=-1
  LTZone : $bdroot/Neuron Elements/LTZone  SystemSampleTime=-1  NM=6  FB=0.7  IT=0.005  T=0.001
  Simple Membrane{,1..8} (9 alike) : $bdroot/Neuron Elements/Simple Membrane  SystemSampleTime=-1  ACm=1e-9  ARm=1e7  ECm=1e-9  ERm=1e7  ARFm=1e8  ERFm=1e8
  Sum1 : Sum  InputSameDT=on  SaturateOnIntegerOverflow=on  OutDataTypeStr=Inherit: Same as first input
  Sum12 : Sum  InputSameDT=on  SaturateOnIntegerOverflow=on  OutDataTypeStr=Inherit: Same as first input
  Sum2 : Sum  Inputs=+++  InputSameDT=on  SaturateOnIntegerOverflow=on  OutDataTypeStr=Inherit: Same as first input
  Sum3 : Sum  Inputs=+++  InputSameDT=on  SaturateOnIntegerOverflow=on  OutDataTypeStr=Inherit: Same as first input
  Sum4 : Sum  Inputs=+++  InputSameDT=on  SaturateOnIntegerOverflow=on  OutDataTypeStr=Inherit: Same as first input
  Sum5 : Sum  InputSameDT=on  SaturateOnIntegerOverflow=on  OutDataTypeStr=Inherit: Same as first input
  Sum7 : Sum  Inputs=++++  InputSameDT=on  SaturateOnIntegerOverflow=on  OutDataTypeStr=Inherit: Same as first input
  Synapse{,1..7} (8 alike) : $bdroot/Neuron Elements/Synapse  SystemSampleTime=-1  SecretionTC=0.001  DecompositionTC=0.01  ksi=2  gamma=1e8
  Out : Outport  VectorParamsAs1DForOutWhenUnconnected=off
  Visual : Outport  Port=2  VectorParamsAs1DForOutWhenUnconnected=off
  Potential : Outport  Port=3  VectorParamsAs1DForOutWhenUnconnected=off
  wires:
  Simple Membrane5/2 -> Sum2/2
  Sum3/1 -> Sum2/3
  C9/1 -> Simple Membrane6/4
  C8/1 -> Simple Membrane6/2
  Simple Membrane6/2 -> Sum3/2
  Simple Membrane6/1 -> Sum3/1
  C5/1 -> Simple Membrane4/4
  C4/1 -> Simple Membrane4/2
  Simple Membrane/1 -> Sum7/2
  Simple Membrane/2 -> Sum7/3
  Sum1/1 -> Sum7/1
  Simple Membrane4/2 -> Sum1/2
  Simple Membrane4/1 -> Sum1/1
  LTZone/1 -> Simple Membrane4/3, Simple Membrane/3, Simple Membrane5/3, Simple Membrane6/3, Simple Membrane7/3, Simple Membrane8/3
  Sum7/1 -> LTZone/1, Potential/1
  Simple Membrane1/2 -> Simple Membrane/4, Sum12/2
  Simple Membrane1/1 -> Simple Membrane/2, Sum12/1
  Arresting1/1 -> Synapse1/1
  Stimulate1/1 -> Synapse/1
  C1/1 -> LTZone/2
  LTZone/3 -> Out/1
  LTZone/2 -> Visual/1
  Simple Membrane2/1 -> Simple Membrane1/2
  Simple Membrane2/2 -> Simple Membrane1/4
  Simple Membrane3/1 -> Simple Membrane2/2
  Simple Membrane3/2 -> Simple Membrane2/4
  Synapse1/1 -> Simple Membrane3/5
  C3/1 -> Simple Membrane3/4
  C2/1 -> Simple Membrane3/2
  Synapse/1 -> Simple Membrane3/1
  Synapse2/1 -> Simple Membrane2/1
  Stimulate2/1 -> Synapse2/1
  Synapse3/1 -> Simple Membrane1/1
  Stimulate3/1 -> Synapse3/1
  Synapse4/1 -> Simple Membrane/1
  Stimulate4/1 -> Synapse4/1
  Arresting2/1 -> Synapse5/1
  Synapse5/1 -> Simple Membrane2/5
  Arresting3/1 -> Synapse6/1
  Synapse6/1 -> Simple Membrane1/5
  Arresting4/1 -> Synapse7/1
  Synapse7/1 -> Simple Membrane/5
  C7/1 -> Simple Membrane5/4
  C6/1 -> Simple Membrane5/2
  Simple Membrane5/1 -> Sum2/1
  Sum2/1 -> Sum7/4
  Simple Membrane7/2 -> Sum4/2
  Sum5/1 -> Sum4/3
  C13/1 -> Simple Membrane8/4
  C12/1 -> Simple Membrane8/2
  Simple Membrane8/2 -> Sum5/2
  Simple Membrane8/1 -> Sum5/1
  C11/1 -> Simple Membrane7/4
  C10/1 -> Simple Membrane7/2
  Simple Membrane7/1 -> Sum4/1
  Sum4/1 -> Sum3/3

== system NeuroModelerLibrary/Support/Electric Engine Model ==
  Voltage : Inport
  Ext moment : Inport  Port=2
  Gain : Gain  Gain=10
  Gain1 : Gain  Gain=10
  Integrator : Integrator
  Integrator1 : Integrator
  Scope : Scope  NumInputPorts=3
  Sum : Sum  Inputs=|+-
  Sum1 : Sum  Inputs=|+-
  Sum2 : Sum  Inputs=|++
  Transfer Fcn : TransferFcn  Denominator=[0.001 0.1]
  Transfer Fcn1 : TransferFcn  Denominator=[10 0]
  Transfer Fcn2 : TransferFcn  Denominator=[10 0]
  Angle : Outport  Tag=Angle  VectorParamsAs1DForOutWhenUnconnected=off
  Speed : Outport  Port=2  VectorParamsAs1DForOutWhenUnconnected=off
  Moment : Outport  Port=3  VectorParamsAs1DForOutWhenUnconnected=off
  wires:
  Voltage/1 -> Sum/1
  Sum/1 -> Transfer Fcn/1
  Transfer Fcn/1 -> Gain/1
  Gain/1 -> Sum1/1, Transfer Fcn2/1, Moment/1
  Sum1/1 -> Transfer Fcn1/1
  Transfer Fcn1/1 -> Integrator/1, Scope/2, Speed/1, Gain1/1
  Gain1/1 -> Sum/2
  Ext moment/1 -> Sum1/2
  Integrator/1 -> Angle/1, Scope/1, Sum2/1
  Transfer Fcn2/1 -> Integrator1/1
  Integrator1/1 -> Sum2/2
  Sum2/1 -> Scope/3

== system NeuroModelerLibrary/Support/Inertial Link ==
  In1 : Inport
  In2 : Inport  Port=2
  Fcn1 : Fcn  Expr=1/u
  Integrator : Integrator
  Product : Product  InputSameDT=on  RndMeth=Zero  SaturateOnIntegerOverflow=on  OutDataTypeStr=Inherit: Same as first input
  Product1 : Product  InputSameDT=on  RndMeth=Zero  SaturateOnIntegerOverflow=on  OutDataTypeStr=Inherit: Same as first input
  Sum : Sum  Inputs=+-  InputSameDT=on  SaturateOnIntegerOverflow=on  OutDataTypeStr=Inherit: Same as first input
  Out1 : Outport  InitialOutput=0  VectorParamsAs1DForOutWhenUnconnected=off
  wires:
  Sum/1 -> Integrator/1
  Product/1 -> Sum/2
  Product1/1 -> Sum/1
  Fcn1/1 -> Product/2, Product1/2
  Integrator/1 -> Product/1, Out1/1
  In1/1 -> Product1/1
  In2/1 -> Fcn1/1

== system NeuroModelerLibrary/Support/Inertial Link With Reset ==
  Value : Inport
  TC : Inport  Port=2
  X0 : Inport  Port=3
  Reset : Inport  Port=4
  Fcn1 : Fcn  Expr=1/u
  Integrator Limited : Integrator  ExternalReset=either  InitialConditionSource=external  UpperSaturationLimit=1  LowerSaturationLimit=0  ShowStatePort=on
  Product : Product  InputSameDT=on  RndMeth=Zero  SaturateOnIntegerOverflow=on  OutDataTypeStr=Inherit: Same as first input
  Product1 : Product  InputSameDT=on  RndMeth=Zero  SaturateOnIntegerOverflow=on  OutDataTypeStr=Inherit: Same as first input
  Sum : Sum  Inputs=+-  InputSameDT=on  SaturateOnIntegerOverflow=on  OutDataTypeStr=Inherit: Same as first input
  Out : Outport  InitialOutput=0  VectorParamsAs1DForOutWhenUnconnected=off
  State : Outport  Port=2  InitialOutput=0  VectorParamsAs1DForOutWhenUnconnected=off
  wires:
  Sum/1 -> Integrator Limited/1
  Product/1 -> Sum/2
  Product1/1 -> Sum/1
  Fcn1/1 -> Product/2, Product1/2
  Integrator Limited/1 -> Product/1, Out/1
  Value/1 -> Product1/1
  TC/1 -> Fcn1/1
  X0/1 -> Integrator Limited/3
  Reset/1 -> Integrator Limited/2
  Integrator Limited/State -> State/1

== system NeuroModelerLibrary/Support/Sign Separator ==
  In1 : Inport
  Abs : Abs
  Compare To Zero : simulink/Logic and Bit Operations/Compare To Zero  relop=>=  OutDataTypeStr=uint8  ZeroCross=off
  Compare To Zero1 : simulink/Logic and Bit Operations/Compare To Zero  relop=<  OutDataTypeStr=uint8  ZeroCross=off
  Product : Product  RndMeth=Zero
  Product1 : Product  RndMeth=Zero
  Sign : Signum
  Sign1 : Signum
  Out1 : Outport  VectorParamsAs1DForOutWhenUnconnected=off
  Out2 : Outport  Port=2  VectorParamsAs1DForOutWhenUnconnected=off
  wires:
  In1/1 -> Product/1, Sign/1, Sign1/1, Abs/1
  Sign/1 -> Compare To Zero/1
  Sign1/1 -> Compare To Zero1/1
  Abs/1 -> Product1/2
  Compare To Zero/1 -> Product/2
  Product1/1 -> Out2/1
  Product/1 -> Out1/1
  Compare To Zero1/1 -> Product1/1

== system NeuroModelerLibrary/Support/Two-output Pulse Generator ==
  Clock : Clock
  Constant : Constant  Value=0
  Discrete Pulse Generator : DiscretePulseGenerator  Amplitude=A  Period=P1  PulseWidth=PW  SampleTime=ST
  Discrete Pulse Generator1 : DiscretePulseGenerator  Amplitude=A  Period=P2  PulseWidth=PW  SampleTime=ST
  Switch : Switch  Threshold=OOff1  SaturateOnIntegerOverflow=on  InputSameDT=on
  Switch1 : Switch  Threshold=OOff2  SaturateOnIntegerOverflow=on  InputSameDT=on
  Transport Delay : TransportDelay  DelayTime=OOn1
  Transport Delay1 : TransportDelay  DelayTime=OOn2
  Out1 : Outport  InitialOutput=0  VectorParamsAs1DForOutWhenUnconnected=off
  Out2 : Outport  Port=2  InitialOutput=0  VectorParamsAs1DForOutWhenUnconnected=off
  wires:
  Switch1/1 -> Out2/1
  Switch/1 -> Out1/1
  Clock/1 -> Switch1/2, Switch/2
  Transport Delay/1 -> Switch/3
  Transport Delay1/1 -> Switch1/3
  Discrete Pulse Generator1/1 -> Transport Delay1/1
  Constant/1 -> Switch1/1, Switch/1
  Discrete Pulse Generator/1 -> Transport Delay/1

== system NeuroModelerLibrary/Classic Models/Alpha-Function Synapse (nonsmooth)/Triggered Subsystem ==
  In1 : Inport
  Trigger : TriggerPort  VariantControl=Variant
  Out1 : Outport
  wires:
  In1/1 -> Out1/1

== system NeuroModelerLibrary/Classic Models/Alpha-Function Synapse (smooth)/Triggered Subsystem ==
  In1 : Inport
  Trigger : TriggerPort  VariantControl=Variant
  Out1 : Outport
  wires:
  In1/1 -> Out1/1

== system NeuroModelerLibrary/Classic Models/IaF Neuron with refractory/Triggered Subsystem ==
  In1 : Inport
  Trigger : TriggerPort  VariantControl=Variant
  Out1 : Outport
  wires:
  In1/1 -> Out1/1

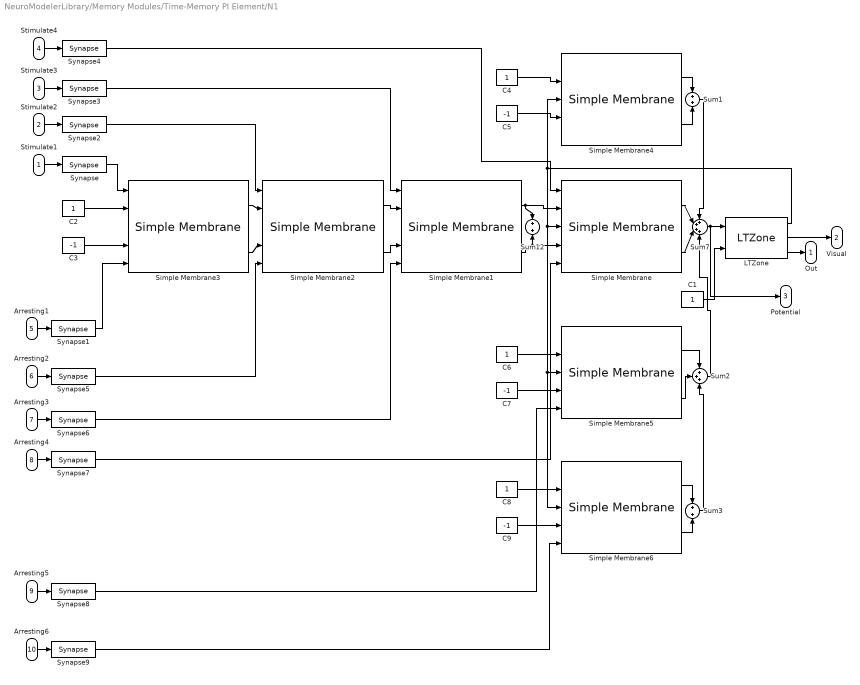
== system NeuroModelerLibrary/Memory Modules/Time-Memory PI Element/N1 ==
  Stimulate1 : Inport
  Stimulate2 : Inport  Port=2
  Stimulate3 : Inport  Port=3
  Stimulate4 : Inport  Port=4
  Arresting1 : Inport  Port=5
  Arresting2 : Inport  Port=6
  Arresting3 : Inport  Port=7
  Arresting4 : Inport  Port=8
  Arresting5 : Inport  Port=9
  Arresting6 : Inport  Port=10
  C{1..2,4,6,8} (5 alike) : Constant
  C{3,5,7,9} (4 alike) : Constant  Value=-1
  LTZone : $bdroot/Neuron Elements/LTZone  NM=4  FB=0.9  IT=0.005  T=0.001
  Simple Membrane{,1..6} (7 alike) : $bdroot/Neuron Elements/Simple Membrane  ACm=1e-9  ARm=1e7  ECm=1e-9  ERm=1e7  ARFm=1e8  ERFm=1e8
  Sum1 : Sum  InputSameDT=on  SaturateOnIntegerOverflow=on  OutDataTypeStr=Inherit: Same as first input
  Sum12 : Sum  InputSameDT=on  SaturateOnIntegerOverflow=on  OutDataTypeStr=Inherit: Same as first input
  Sum2 : Sum  Inputs=+++  InputSameDT=on  SaturateOnIntegerOverflow=on  OutDataTypeStr=Inherit: Same as first input
  Sum3 : Sum  InputSameDT=on  SaturateOnIntegerOverflow=on  OutDataTypeStr=Inherit: Same as first input
  Sum7 : Sum  Inputs=++++  InputSameDT=on  SaturateOnIntegerOverflow=on  OutDataTypeStr=Inherit: Same as first input
  Synapse{,1..9} (10 alike) : $bdroot/Neuron Elements/Synapse  SecretionTC=0.001  DecompositionTC=0.01  ksi=2  gamma=1e8
  Out : Outport  VectorParamsAs1DForOutWhenUnconnected=off
  Visual : Outport  Port=2  VectorParamsAs1DForOutWhenUnconnected=off
  Potential : Outport  Port=3  VectorParamsAs1DForOutWhenUnconnected=off
  wires:
  Simple Membrane5/2 -> Sum2/2
  Sum3/1 -> Sum2/3
  C9/1 -> Simple Membrane6/4
  C8/1 -> Simple Membrane6/2
  Simple Membrane6/2 -> Sum3/2
  Simple Membrane6/1 -> Sum3/1
  C5/1 -> Simple Membrane4/4
  C4/1 -> Simple Membrane4/2
  Simple Membrane/1 -> Sum7/2
  Simple Membrane/2 -> Sum7/3
  Sum1/1 -> Sum7/1
  Simple Membrane4/2 -> Sum1/2
  Simple Membrane4/1 -> Sum1/1
  LTZone/1 -> Simple Membrane4/3, Simple Membrane/3, Simple Membrane6/3, Simple Membrane5/3
  Sum7/1 -> Potential/1, LTZone/1
  Simple Membrane1/2 -> Simple Membrane/4, Sum12/2
  Simple Membrane1/1 -> Simple Membrane/2, Sum12/1
  Arresting1/1 -> Synapse1/1
  Stimulate1/1 -> Synapse/1
  C1/1 -> LTZone/2
  LTZone/3 -> Out/1
  LTZone/2 -> Visual/1
  Simple Membrane2/1 -> Simple Membrane1/2
  Simple Membrane2/2 -> Simple Membrane1/4
  Simple Membrane3/1 -> Simple Membrane2/2
  Simple Membrane3/2 -> Simple Membrane2/4
  Synapse1/1 -> Simple Membrane3/5
  C3/1 -> Simple Membrane3/4
  C2/1 -> Simple Membrane3/2
  Synapse/1 -> Simple Membrane3/1
  Synapse2/1 -> Simple Membrane2/1
  Stimulate2/1 -> Synapse2/1
  Synapse3/1 -> Simple Membrane1/1
  Stimulate3/1 -> Synapse3/1
  Synapse4/1 -> Simple Membrane/1
  Stimulate4/1 -> Synapse4/1
  Arresting2/1 -> Synapse5/1
  Synapse5/1 -> Simple Membrane2/5
  Arresting3/1 -> Synapse6/1
  Synapse6/1 -> Simple Membrane1/5
  Arresting4/1 -> Synapse7/1
  Synapse7/1 -> Simple Membrane/5
  C7/1 -> Simple Membrane5/4
  C6/1 -> Simple Membrane5/2
  Simple Membrane5/1 -> Sum2/1
  Sum2/1 -> Sum7/4
  Arresting5/1 -> Synapse8/1
  Synapse8/1 -> Simple Membrane5/5
  Arresting6/1 -> Synapse9/1
  Synapse9/1 -> Simple Membrane6/5

== system NeuroModelerLibrary/Neuron Elements/CSNM Synapse-D/Triggered Subsystem ==
  In1 : Inport
  Trigger : TriggerPort  VariantControl=Variant
  Out1 : Outport
  wires:
  In1/1 -> Out1/1

== system NeuroModelerLibrary/Neuron Elements/Ion System v0.1/Inertial Link (H1) ==
  In1 : Inport
  In2 : Inport  Port=2
  Fcn1 : Fcn  Expr=1/u
  Integrator : Integrator
  Product : Product  InputSameDT=on  RndMeth=Zero  SaturateOnIntegerOverflow=on  OutDataTypeStr=Inherit: Same as first input
  Product1 : Product  InputSameDT=on  RndMeth=Zero  SaturateOnIntegerOverflow=on  OutDataTypeStr=Inherit: Same as first input
  Sum : Sum  Inputs=+-  InputSameDT=on  SaturateOnIntegerOverflow=on  OutDataTypeStr=Inherit: Same as first input
  Out1 : Outport  InitialOutput=0  VectorParamsAs1DForOutWhenUnconnected=off
  wires:
  Sum/1 -> Integrator/1
  Product/1 -> Sum/2
  Product1/1 -> Sum/1
  Fcn1/1 -> Product/2, Product1/2
  Integrator/1 -> Product/1, Out1/1
  In1/1 -> Product1/1
  In2/1 -> Fcn1/1

== system NeuroModelerLibrary/Neuron Elements/LTZone v0.1/Inertial Link (H1) ==
  In1 : Inport
  In2 : Inport  Port=2
  Fcn1 : Fcn  Expr=1/u
  Integrator : Integrator
  Product : Product  InputSameDT=on  RndMeth=Zero  SaturateOnIntegerOverflow=on  OutDataTypeStr=Inherit: Same as first input
  Product1 : Product  InputSameDT=on  RndMeth=Zero  SaturateOnIntegerOverflow=on  OutDataTypeStr=Inherit: Same as first input
  Sum : Sum  Inputs=+-  InputSameDT=on  SaturateOnIntegerOverflow=on  OutDataTypeStr=Inherit: Same as first input
  Out1 : Outport  InitialOutput=0  VectorParamsAs1DForOutWhenUnconnected=off
  wires:
  In2/1 -> Fcn1/1
  In1/1 -> Product1/1
  Integrator/1 -> Out1/1, Product/1
  Fcn1/1 -> Product1/2, Product/2
  Product1/1 -> Sum/1
  Product/1 -> Sum/2
  Sum/1 -> Integrator/1

== system NeuroModelerLibrary/Neuron Elements/Synapse Ion System v0.1/Inertial Link (H1) ==
  In1 : Inport
  In2 : Inport  Port=2
  Fcn1 : Fcn  Expr=1/u
  Integrator : Integrator
  Product : Product  InputSameDT=on  RndMeth=Zero  SaturateOnIntegerOverflow=on  OutDataTypeStr=Inherit: Same as first input
  Product1 : Product  InputSameDT=on  RndMeth=Zero  SaturateOnIntegerOverflow=on  OutDataTypeStr=Inherit: Same as first input
  Sum : Sum  Inputs=+-  InputSameDT=on  SaturateOnIntegerOverflow=on  OutDataTypeStr=Inherit: Same as first input
  Out1 : Outport  InitialOutput=0  VectorParamsAs1DForOutWhenUnconnected=off
  wires:
  In2/1 -> Fcn1/1
  In1/1 -> Product1/1
  Integrator/1 -> Out1/1, Product/1
  Fcn1/1 -> Product1/2, Product/2
  Product1/1 -> Sum/1
  Product/1 -> Sum/2
  Sum/1 -> Integrator/1

== system NeuroModelerLibrary/Neuron Elements/Synapse v0.1/Inertial Link (H1)1 ==
  In1 : Inport
  In2 : Inport  Port=2
  Fcn1 : Fcn  Expr=1/u
  Integrator : Integrator
  Product : Product  InputSameDT=on  RndMeth=Zero  SaturateOnIntegerOverflow=on  OutDataTypeStr=Inherit: Same as first input
  Product1 : Product  InputSameDT=on  RndMeth=Zero  SaturateOnIntegerOverflow=on  OutDataTypeStr=Inherit: Same as first input
  Sum : Sum  Inputs=+-  InputSameDT=on  SaturateOnIntegerOverflow=on  OutDataTypeStr=Inherit: Same as first input
  Out1 : Outport  InitialOutput=0  VectorParamsAs1DForOutWhenUnconnected=off
  wires:
  In2/1 -> Fcn1/1
  In1/1 -> Product1/1
  Integrator/1 -> Out1/1, Product/1
  Fcn1/1 -> Product1/2, Product/2
  Product1/1 -> Sum/1
  Product/1 -> Sum/2
  Sum/1 -> Integrator/1
